simulink model "fixedVsVariable"  (R2022b)
settings: Solver=VariableStepDiscrete  StartTime=0.0  StopTime=20.0  RelTol=1e-3
settings Model: Creator=gchandra  LastModifiedBy=bensweet
settings SolverCC: AlgebraicLoopSolver=TrustRegion
settings DataIOCC: LimitDataPoints=on  SaveFormat=Array  ReturnWorkspaceOutputs=off  SignalLoggingName=sigsOut
settings OptimizationCC: ExpressionDepthLimit=2147483647  InitFltsAndDblsToZero=on  LifeSpan=inf
settings DebuggingCC: UnconnectedInputMsg=warning  UnconnectedOutputMsg=warning  UnconnectedLineMsg=warning  PregeneratedLibrarySubsystemCodeDiagnostic=none  SFMachineParentedDataDiag=warning
settings HardwareCC: ProdBitPerPointer=32  ProdBitPerSizeT=32  ProdBitPerPtrDiffT=32  ProdLargestAtomicFloat=None  ProdIntDivRoundTo=Undefined  ProdEndianess=Unspecified  ProdWordSize=32  ProdHWDeviceType=32-bit Generic  TargetUnknown=on
settings ModelReferenceCC: EnableRefExpFcnMdlSchedulingChecks=on  PropagateSignalLabelsOutOfModel=off
settings SFSimCC: SimUseLocalCustomCode=off
settings RTWCC: RTWUseLocalCustomCode=off  DLArmComputeVersion=19.05
settings CodeAppCC: StateflowObjectComments=on
settings GRTTargetCC: TargetFcnLib=ansi_tfl_tmw.mat  TargetLangStandard=C89/C90 (ANSI)  CombineOutputUpdateFcns=off  GRTInterface=on
settings ConfigComp: CovMetricSettings=dw  CovSaveCumulativeToWorkspaceVar=on  CovSaveSingleToWorkspaceVar=on  CovExternalEMLEnable=off  CovSFcnEnable=off

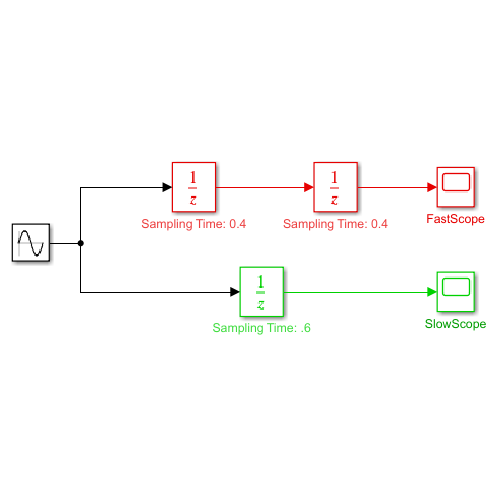
[thumbnail: Simulink's stored preview of the top-level diagram]
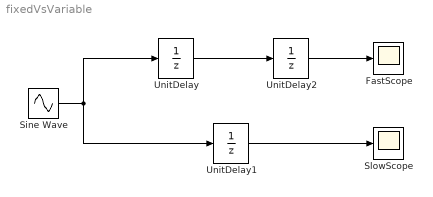
== system fixedVsVariable ==
  FastScope : Scope
  Sine Wave : Sin  SampleTime=0
  SlowScope : Scope
  UnitDelay : UnitDelay  SampleTime=0.4  HasFrameUpgradeWarning=on
      settings: AttributesFormatString=Sampling Time: %<SampleTime>
  UnitDelay1 : UnitDelay  SampleTime=.6  HasFrameUpgradeWarning=on
      settings: AttributesFormatString=Sampling Time: %<SampleTime>
  UnitDelay2 : UnitDelay  SampleTime=0.4  HasFrameUpgradeWarning=on
      settings: AttributesFormatString=Sampling Time: %<SampleTime>
  wires:
  Sine Wave/1 -> UnitDelay/1, UnitDelay1/1
  UnitDelay/1 -> UnitDelay2/1
  UnitDelay2/1 -> FastScope/1
  UnitDelay1/1 -> SlowScope/1
